simulink model "buck_closed_loop_load"  (Simulink 4.0)
settings: Solver=ode45  StartTime=0.0  StopTime=0.003  MaxStep=0.1e-6  RelTol=1e-3
libraries: simulink x1
settings Model: LastModifiedBy=Dragan Maksimovic  BooleanDataType=on

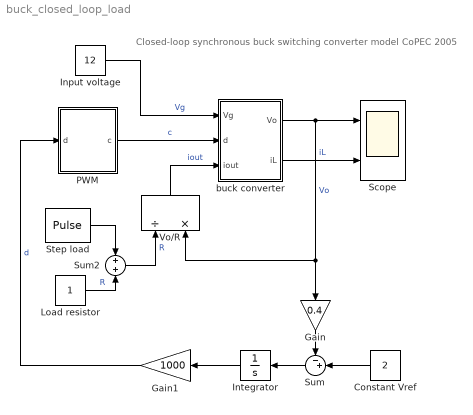
== system buck_closed_loop_load ==
  note: Closed-loop synchronous buck switching converter model
      | CoPEC 2005
  Constant Vref : Constant  Orientation=left  Value=2
  Gain : Gain  Orientation=down  Gain=0.4  Multiplication=Element-wise(K.*u)  SaturateOnIntegerOverflow=on
  Gain1 : Gain  Orientation=left  Gain=1000  Multiplication=Element-wise(K.*u)  SaturateOnIntegerOverflow=on
  Input voltage : Constant  Value=12
  Integrator : Integrator  Orientation=left  ExternalReset=none  InitialConditionSource=internal  InitialCondition=0  LimitOutput=off  UpperSaturationLimit=inf  LowerSaturationLimit=-inf  ShowSaturationPort=off  ShowStatePort=off  AbsoluteTolerance=auto
  Load resistor : Constant  Value=1
  PWM : Subsystem  SimViewingDevice=off
      settings: Permissions=ReadWrite  RTWFcnNameOpts=Auto  RTWFileNameOpts=Auto
  Scope : Scope  NumInputPorts=2
      settings: TimeRange=0.003  YMin=4.9~0  YMax=5.1~10  SaveToWorkspace=off  SaveName=ScopeData  MaxDataPoints=5000
  Step load : DiscretePulseGenerator  PulseType=Time-based  Amplitude=1  Period=0.002  PulseWidth=50  PhaseDelay=0  SampleTime=1
  Sum : Sum  Orientation=left  Inputs=-+|  SaturateOnIntegerOverflow=on
  Sum2 : Sum  Inputs=+|+  SaturateOnIntegerOverflow=on
  Vo/R : Product  Orientation=up  Inputs=/*  Multiplication=Element-wise(.*)  SaturateOnIntegerOverflow=on
  buck converter : Subsystem  SimViewingDevice=off
      settings: Permissions=ReadWrite  RTWFcnNameOpts=Auto  RTWFileNameOpts=Auto
  wires:
  Input voltage/1 -> buck converter/1(Vg)  "Vg"
  buck converter/1(Vo) -> Scope/1, Vo/R/2, Gain/1  "Vo"
  buck converter/2(iL) -> Scope/2  "iL"
  PWM/1(c) -> buck converter/2(d)  "c"
  Vo/R/1 -> buck converter/3(iout)  "iout"
  Gain/1 -> Sum/1
  Constant Vref/1 -> Sum/2
  Sum/1 -> Integrator/1
  Integrator/1 -> Gain1/1
  Gain1/1 -> PWM/1(d)  "d"
  Step load/1 -> Sum2/1
  Load resistor/1 -> Sum2/2  "R"
  Sum2/1 -> Vo/R/1  "R"

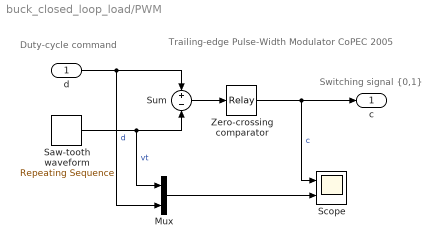
== system buck_closed_loop_load/PWM ==
  note: Duty-cycle
      | command
  note: Switching signal {0,1}
  note: Trailing-edge Pulse-Width Modulator
      | CoPEC 2005
  d : Inport  Port=1  PortDimensions=-1  SampleTime=-1  DataType=auto
      settings: SignalType=auto
  Mux : Mux  Inputs=2
  Saw-tooth waveform : simulink/Sources/Repeating Sequence  rep_seq_t=[0 0.001e-5 1e-5]  rep_seq_y=[1 0 1]
  Scope : Scope  NumInputPorts=2
      settings: TimeRange=auto  YMin=0~0  YMax=1.5~1.5  SaveToWorkspace=off  MaxDataPoints=5000
  Sum : Sum  Inputs=+|-  SaturateOnIntegerOverflow=on
  Zero-crossing comparator : Relay  OnSwitchValue=eps  OffSwitchValue=eps  OnOutputValue=1  OffOutputValue=0
  c : Outport  Port=1
  wires:
  Saw-tooth waveform/1 -> Mux/1, Sum/2  "vt"
  d/1 -> Mux/2, Sum/1  "d"
  Zero-crossing comparator/1 -> c/1, Scope/1  "c"
  Sum/1 -> Zero-crossing comparator/1
  Mux/1 -> Scope/2

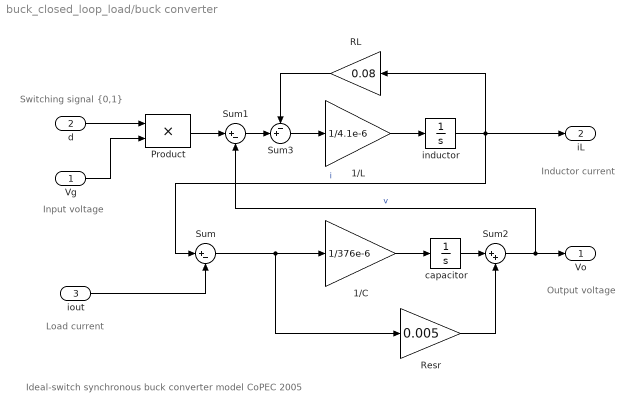
== system buck_closed_loop_load/buck converter ==
  note: Load current
  note: Input voltage
  note: Inductor current
  note: Output voltage
  note: Switching signal {0,1}
  note: Ideal-switch synchronous buck converter model
      | CoPEC 2005
  Vg : Inport  Port=1  PortDimensions=-1  SampleTime=-1  DataType=auto
      settings: SignalType=auto
  d : Inport  Port=2  PortDimensions=-1  SampleTime=-1  DataType=auto
      settings: SignalType=auto
  iout : Inport  Port=3  PortDimensions=-1  SampleTime=-1  DataType=auto
      settings: SignalType=auto
  1/C : Gain  Gain=1/376e-6  Multiplication=Element-wise(K.*u)  SaturateOnIntegerOverflow=on
  1/L : Gain  Gain=1/4.1e-6  Multiplication=Element-wise(K.*u)  SaturateOnIntegerOverflow=on
  Product : Product  Inputs=2  Multiplication=Element-wise(.*)  SaturateOnIntegerOverflow=on
  RL : Gain  Orientation=left  Gain=0.08  Multiplication=Element-wise(K.*u)  SaturateOnIntegerOverflow=on
  Resr : Gain  Gain=0.005  Multiplication=Element-wise(K.*u)  SaturateOnIntegerOverflow=on
  Sum : Sum  Inputs=|+-  SaturateOnIntegerOverflow=on
  Sum1 : Sum  Inputs=|+-  SaturateOnIntegerOverflow=on
  Sum2 : Sum  Inputs=|++  SaturateOnIntegerOverflow=on
  Sum3 : Sum  Inputs=-+|  SaturateOnIntegerOverflow=on
  capacitor : Integrator  ExternalReset=none  InitialConditionSource=internal  InitialCondition=0  LimitOutput=off  UpperSaturationLimit=inf  LowerSaturationLimit=-inf  ShowSaturationPort=off  ShowStatePort=off  AbsoluteTolerance=auto
  inductor : Integrator  ExternalReset=none  InitialConditionSource=internal  InitialCondition=0  LimitOutput=off  UpperSaturationLimit=inf  LowerSaturationLimit=-inf  ShowSaturationPort=off  ShowStatePort=off  AbsoluteTolerance=auto
  Vo : Outport  Port=1
  iL : Outport  Port=2
  wires:
  iout/1 -> Sum/2
  d/1 -> Product/1
  Resr/1 -> Sum2/2
  capacitor/1 -> Sum2/1
  Sum3/1 -> 1/L/1
  RL/1 -> Sum3/1
  Sum1/1 -> Sum3/2
  Sum2/1 -> Sum1/2, Vo/1  "v"
  Product/1 -> Sum1/1
  inductor/1 -> Sum/1, RL/1, iL/1  "i"
  1/L/1 -> inductor/1
  Sum/1 -> 1/C/1, Resr/1
  1/C/1 -> capacitor/1
  Vg/1 -> Product/2
